simulink model "satellite_attitude_kalman_model"  (R2017a)
settings: Solver=VariableStepAuto  StartTime=0.0  StopTime=tdur  FixedStep=dt  RelTol=1e-3
values from neighbouring files (symbols this model uses):
  Ad_b = expm(A_b*dt)    [linear_eq.m]
  Ad_rw = sysd_rw.a    [satellite_attitude_kalman_run.m]
  b = 0.000178    [satellite_attitude_kalman_run.m]
  Bd_b = integral(fun,0,dt,'ArrayValued',true)*B_b    [linear_eq.m]
  Bd_rw = sysd_rw.b    [satellite_attitude_kalman_run.m]
  C_lqe = [ 0 0 0 0 0 0 ... (first row only)    [satellite_attitude_kalman_run.m]
  Cd_rw = sysd_rw.c    [satellite_attitude_kalman_run.m]
  DCM_b_i_0 = eul2qua(x_pos_init,y_pos_init,z_pos_init)    [satellite_attitude_kalman_run.m]
  DCM_b_w = [ 0.40825 0.40825 -0.81650 ... (first row only)    [satellite_attitude_kalman_run.m]
  dt_c = 0.05    [satellite_attitude_kalman_run.m]
  dt_w = 0.05    [satellite_attitude_kalman_run.m]
  grav_ref = [0 ; 0 ; -1]    [satellite_attitude_kalman_run.m]
  grav_variance = 0    [satellite_attitude_kalman_run.m]
  i_0 = [0 ;0 ;0]    [satellite_attitude_kalman_run.m]
  I_b = diag([Ixx Iyy Izz])    [satellite_attitude_kalman_run.m]
  I_w = diag([Ia Ia Ia])    [satellite_attitude_kalman_run.m]
  J = 0.00725    [satellite_attitude_kalman_run.m]
  K_e = 0.071    [satellite_attitude_kalman_run.m]
  K_t = 0.070    (= 0.07)    [satellite_attitude_kalman_run.m]
  Kd = 1.5    [satellite_attitude_kalman_run.m]
  Kp = dlqr(Ad_b,Bd_b,Q_lqr,R_lqr)    [satellite_attitude_kalman_run.m]
  L = 0.00339    [satellite_attitude_kalman_run.m]
  Lss = dlqe(Ad_b, eye(6,6),C_lqe, Q_lqe,R_lqe)    [satellite_attitude_kalman_run.m]
  mag_ref = [0 ; 1400 ; 0]    [satellite_attitude_kalman_run.m]
  mag_variance = [0;0;0]    [satellite_attitude_kalman_run.m]
  omega_0 = [x_rate_init ;y_rate_init ;z_rate_init]    [satellite_attitude_kalman_run.m]
  omega_variance = [0;0;0]    [satellite_attitude_kalman_run.m]
  R = 1.52    [satellite_attitude_kalman_run.m]
  speed_0 = [RW1_init ;RW2_init ;RW3_init]    [satellite_attitude_kalman_run.m]
  theta_0 = [x_pos_init ;y_pos_init ;z_pos_init]    [satellite_attitude_kalman_run.m]
  v_max = 10    [satellite_attitude_kalman_run.m]
undefined symbols (not defined in the file or in its folder): DiscIntNeverNeededParam
libraries: simulink x20, vrlib x6, dspinverses x3
settings Model: Creator=Goh  LastModifiedBy=Rusty Goh
settings SolverCC: MaxConsecutiveMinStep=2

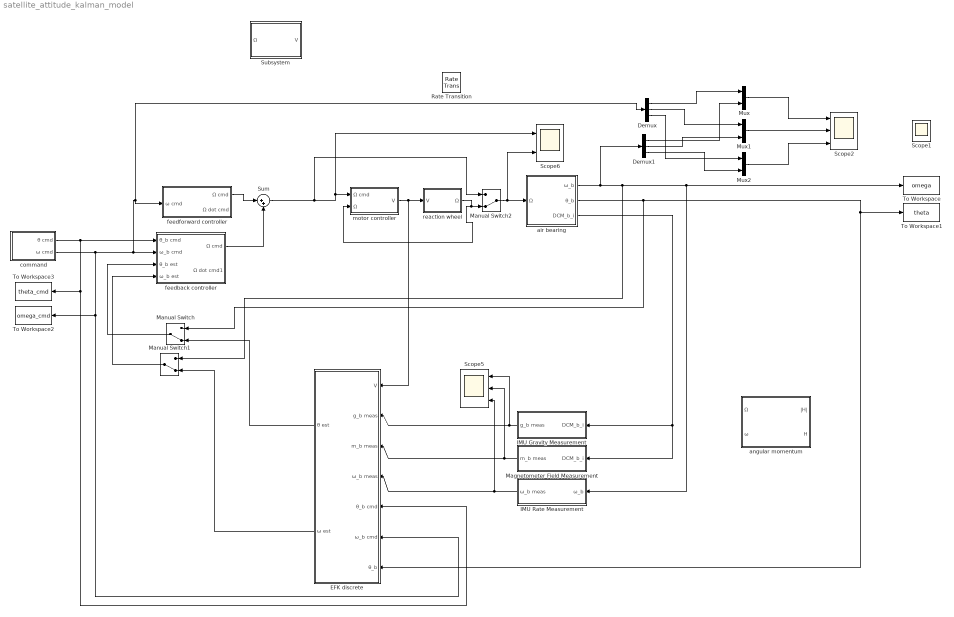
== system satellite_attitude_kalman_model ==
  Demux : Demux  Outputs=3
  Demux1 : Demux  Outputs=3
  EFK discrete : Subsystem
  IMU Gravity Measurement : Subsystem
  IMU Rate Measurement : Subsystem
  Magnetometer Field Measurement : Subsystem
  Manual Switch : ManualSwitch  CurrentSetting=0
  Manual Switch1 : ManualSwitch  CurrentSetting=0
  Manual Switch2 : ManualSwitch  CurrentSetting=0
  Mux : Mux  Inputs=2
  Mux1 : Mux  Inputs=2
  Mux2 : Mux  Inputs=2
  Rate Transition : RateTransition
  Scope1 : Scope  NumInputPorts=3
  Scope2 : Scope  NumInputPorts=3
  Scope5 : Scope  NumInputPorts=3
  Scope6 : Scope  NumInputPorts=2
  Subsystem : Subsystem  mask{Kc=1, Kp=75, Ki=1, Kd=1}
  Sum : Sum  Inputs=|++
  To Workspace : ToWorkspace  VariableName=omega  SampleTime=-1
  To Workspace1 : ToWorkspace  VariableName=theta  SampleTime=-1
  To Workspace2 : ToWorkspace  VariableName=omega_cmd  SaveFormat=Timeseries  SampleTime=-1
  To Workspace3 : ToWorkspace  VariableName=theta_cmd  SaveFormat=Timeseries  SampleTime=-1
  air bearing : Subsystem
  angular momentum : Subsystem
  command : Subsystem
  feedback controller : Subsystem
  feedforward controller : Subsystem
  motor controller : Subsystem
  reaction wheel : Subsystem
  wires:
  Magnetometer Field Measurement/1(m_b meas) -> Scope5/2, EFK discrete/3(m_b meas)
  IMU Rate Measurement/1(ω_b meas) -> Scope5/3, EFK discrete/4(ω_b meas)
  IMU Gravity Measurement/1(g_b meas) -> Scope5/1, EFK discrete/2(g_b meas)
  command/1(θ cmd) -> To Workspace3/1, EFK discrete/5(θ_b cmd), feedback controller/1(θ_b cmd)
  feedback controller/1(Ω cmd) -> Sum/2
  command/2(ω cmd) -> To Workspace2/1, EFK discrete/6(ω_b cmd), Demux/1, feedforward controller/1(ω cmd), feedback controller/2(ω_b cmd)
  air bearing/2(θ_b) -> Manual Switch/1, To Workspace1/1, EFK discrete/7("θ_b ")
  feedforward controller/1(Ω cmd) -> Sum/1
  Mux/1 -> Scope2/1
  Mux1/1 -> Scope2/2
  Mux2/1 -> Scope2/3
  Demux/1 -> Mux/1
  Demux1/1 -> Mux/2
  Demux/2 -> Mux1/1
  Demux1/2 -> Mux1/2
  Demux/3 -> Mux2/1
  Demux1/3 -> Mux2/2
  air bearing/3(DCM_b_i) -> Magnetometer Field Measurement/1(DCM_b_i), IMU Gravity Measurement/1(DCM_b_i)
  EFK discrete/2(ω est) -> Manual Switch1/2
  air bearing/1(ω_b) -> Demux1/1, Manual Switch1/1, IMU Rate Measurement/1(ω_b), To Workspace/1
  EFK discrete/1(θ est) -> Manual Switch/2
  Manual Switch/1 -> feedback controller/3(θ_b est)
  Manual Switch1/1 -> feedback controller/4(ω_b est)
  motor controller/1(V) -> EFK discrete/1(V), reaction wheel/1(V)
  Manual Switch2/1 -> Scope6/2, air bearing/1(Ω)
  reaction wheel/1(Ω) -> Manual Switch2/2, motor controller/2(Ω)
  Sum/1 -> Manual Switch2/1, motor controller/1(Ω cmd), Scope6/1

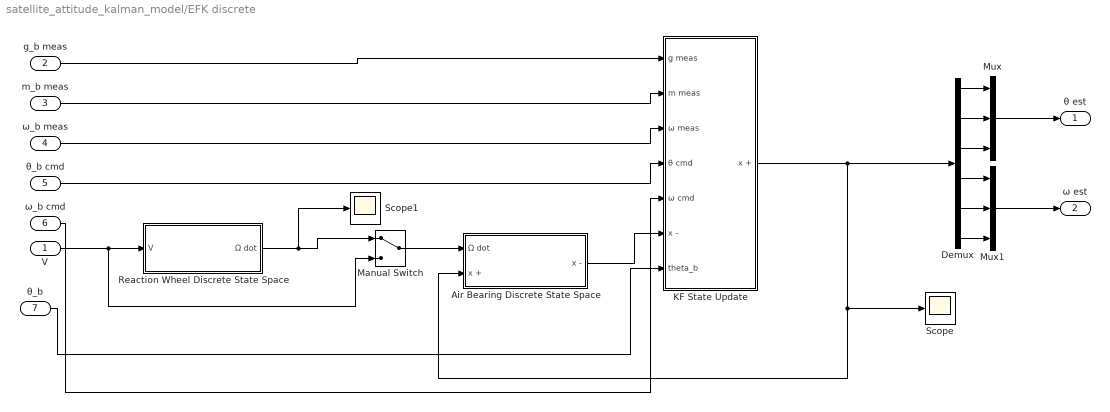
== system satellite_attitude_kalman_model/EFK discrete ==
  V : Inport
  g_b meas : Inport  Port=2
  m_b meas : Inport  Port=3
  ω_b meas : Inport  Port=4
  θ_b cmd : Inport  Port=5
  ω_b cmd : Inport  Port=6
  "θ_b " : Inport  Port=7
  Air Bearing Discrete State Space : Subsystem
  Demux : Demux  Outputs=6
  KF State Update : Subsystem
  Manual Switch : ManualSwitch
  Mux : Mux  Inputs=3
  Mux1 : Mux  Inputs=3
  Reaction Wheel Discrete State Space : Subsystem
  Scope : Scope
  Scope1 : Scope
  θ est : Outport
  ω est : Outport  Port=2
  wires:
  g_b meas/1 -> KF State Update/1(g meas)
  m_b meas/1 -> KF State Update/2(m meas)
  ω_b meas/1 -> KF State Update/3(ω meas)
  θ_b cmd/1 -> KF State Update/4(θ cmd)
  ω_b cmd/1 -> KF State Update/5(ω cmd)
  Air Bearing Discrete State Space/1(x -) -> KF State Update/6(x -)
  Demux/2 -> Mux/2
  Demux/1 -> Mux/1
  Demux/3 -> Mux/3
  Demux/4 -> Mux1/1
  Demux/5 -> Mux1/2
  Demux/6 -> Mux1/3
  Mux/1 -> θ est/1
  Mux1/1 -> ω est/1
  "θ_b "/1 -> KF State Update/7(theta_b)
  KF State Update/1(x +) -> Air Bearing Discrete State Space/2(x +), Scope/1, Demux/1
  V/1 -> Reaction Wheel Discrete State Space/1(V), Manual Switch/2
  Manual Switch/1 -> Air Bearing Discrete State Space/1(Ω dot)
  Reaction Wheel Discrete State Space/1(Ω dot) -> Scope1/1, Manual Switch/1

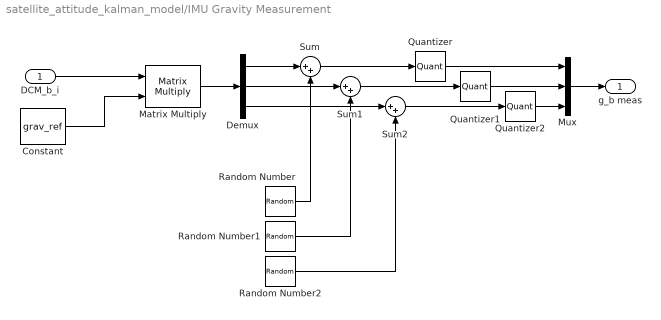
== system satellite_attitude_kalman_model/IMU Gravity Measurement ==
  DCM_b_i : Inport
  Constant : Constant  Value=grav_ref  VectorParams1D=off
  Demux : Demux  Outputs=3
  Matrix Multiply : Product  Multiplication=Matrix(*)
  Mux : Mux  Inputs=3
  Quantizer : Quantizer  QuantizationInterval=0.01
  Quantizer1 : Quantizer  QuantizationInterval=0.01
  Quantizer2 : Quantizer  QuantizationInterval=0.01
  Random Number : RandomNumber  Variance=grav_variance  SampleTime=dt_c
  Random Number1 : RandomNumber  Variance=grav_variance  SampleTime=dt_c
  Random Number2 : RandomNumber  Variance=grav_variance  SampleTime=dt_c
  Sum : Sum  Inputs=|++
  Sum1 : Sum  Inputs=|++
  Sum2 : Sum  Inputs=|++
  g_b meas : Outport
  wires:
  Demux/1 -> Sum/1
  Demux/2 -> Sum1/1
  Demux/3 -> Sum2/1
  Sum2/1 -> Quantizer2/1
  Sum1/1 -> Quantizer1/1
  Sum/1 -> Quantizer/1
  Random Number/1 -> Sum/2
  Random Number1/1 -> Sum1/2
  Random Number2/1 -> Sum2/2
  Mux/1 -> g_b meas/1
  DCM_b_i/1 -> Matrix Multiply/1
  Constant/1 -> Matrix Multiply/2
  Matrix Multiply/1 -> Demux/1
  Quantizer/1 -> Mux/1
  Quantizer1/1 -> Mux/2
  Quantizer2/1 -> Mux/3

== system satellite_attitude_kalman_model/IMU Rate Measurement ==
  ω_b : Inport
  Demux : Demux  Outputs=3
  Mux : Mux  Inputs=3
  Random Number : RandomNumber  Variance=omega_variance(1)  SampleTime=dt_c
  Random Number1 : RandomNumber  Variance=omega_variance(2)  SampleTime=dt_c
  Random Number2 : RandomNumber  Variance=omega_variance(3)  SampleTime=dt_c
  Sum : Sum  Inputs=|++
  Sum1 : Sum  Inputs=|++
  Sum2 : Sum  Inputs=|++
  Zero-Order Hold : ZeroOrderHold  SampleTime=dt_c
  ω_b meas : Outport
  wires:
  Demux/1 -> Sum/1
  Demux/2 -> Sum1/1
  Demux/3 -> Sum2/1
  Sum2/1 -> Mux/3
  Sum1/1 -> Mux/2
  Sum/1 -> Mux/1
  Random Number/1 -> Sum/2
  Random Number1/1 -> Sum1/2
  Random Number2/1 -> Sum2/2
  Mux/1 -> ω_b meas/1
  ω_b/1 -> Zero-Order Hold/1
  Zero-Order Hold/1 -> Demux/1

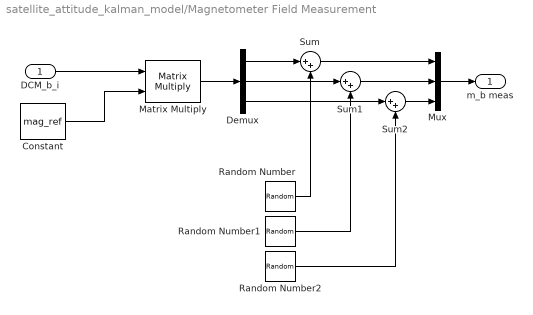
== system satellite_attitude_kalman_model/Magnetometer Field Measurement ==
  DCM_b_i : Inport
  Constant : Constant  Value=mag_ref  VectorParams1D=off
  Demux : Demux  Outputs=3
  Matrix Multiply : Product  Multiplication=Matrix(*)
  Mux : Mux  Inputs=3
  Random Number : RandomNumber  Variance=mag_variance(1)  SampleTime=dt_c
  Random Number1 : RandomNumber  Variance=mag_variance(2)  SampleTime=dt_c
  Random Number2 : RandomNumber  Variance=mag_variance(3)  SampleTime=dt_c
  Sum : Sum  Inputs=|++
  Sum1 : Sum  Inputs=|++
  Sum2 : Sum  Inputs=|++
  m_b meas : Outport
  wires:
  Demux/1 -> Sum/1
  Demux/2 -> Sum1/1
  Demux/3 -> Sum2/1
  Sum2/1 -> Mux/3
  Sum1/1 -> Mux/2
  Sum/1 -> Mux/1
  Random Number/1 -> Sum/2
  Random Number1/1 -> Sum1/2
  Random Number2/1 -> Sum2/2
  Mux/1 -> m_b meas/1
  DCM_b_i/1 -> Matrix Multiply/1
  Constant/1 -> Matrix Multiply/2
  Matrix Multiply/1 -> Demux/1

== system satellite_attitude_kalman_model/Subsystem ==
  Ω : Inport
  Discrete Derivative : simulink/Discrete/Discrete Derivative  gainval=1.0  ICPrevScaledInput=0.0  OutMin=[]  OutMax=[]  OutDataType=fixdt(1, 16)  OutScaling=2^-10  DoSatur=off
  Discrete-Time Integrator : DiscreteIntegrator  InitialConditionSetting=State (most efficient)  SampleTime=-1  ICPrevOutput=DiscIntNeverNeededParam  ICPrevScaledInput=DiscIntNeverNeededParam
  Kc : Gain  Gain=Kc  SaturateOnIntegerOverflow=on  OutDataTypeStr=Inherit: Same as input  ParamDataTypeStr=Inherit: Same as input
  Kd : Gain  Gain=Kd  SaturateOnIntegerOverflow=on  OutDataTypeStr=Inherit: Same as input  ParamDataTypeStr=Inherit: Same as input
  Ki : Gain  Gain=Ki  SaturateOnIntegerOverflow=on  OutDataTypeStr=Inherit: Same as input  ParamDataTypeStr=Inherit: Same as input
  Kp : Gain  Gain=Kp  SaturateOnIntegerOverflow=on  OutDataTypeStr=Inherit: Same as input  ParamDataTypeStr=Inherit: Same as input
  Sum1 : Sum  Inputs=+++
  V : Outport
  wires:
  Ki/1 -> Discrete-Time Integrator/1
  Kc/1 -> Ki/1, Kp/1, Kd/1
  Sum1/1 -> V/1
  Kd/1 -> Discrete Derivative/1
  Discrete Derivative/1 -> Sum1/1
  Kp/1 -> Sum1/2
  Discrete-Time Integrator/1 -> Sum1/3
  Ω/1 -> Kc/1

== system satellite_attitude_kalman_model/air bearing ==
  Ω : Inport
  Integrator : Integrator  InitialCondition=omega_0
  Integrator1 : Integrator  InitialCondition=theta_0
  air bearing dyamics : Subsystem
  ω to DCM : Subsystem
  ω_b : Outport
  θ_b : Outport  Port=2
  DCM_b_i : Outport  Port=3
  wires:
  Ω/1 -> air bearing dyamics/1(Ω_w)
  air bearing dyamics/1(ω_dot) -> Integrator/1
  Integrator/1 -> ω to DCM/1(ω), ω_b/1, Integrator1/1, air bearing dyamics/2(ω_b)
  Integrator1/1 -> θ_b/1
  ω to DCM/1(DCM_b_i) -> DCM_b_i/1

== system satellite_attitude_kalman_model/angular momentum ==
  Ω : Inport
  ω : Inport  Port=2
  |H| : Outport
  H : Outport  Port=2

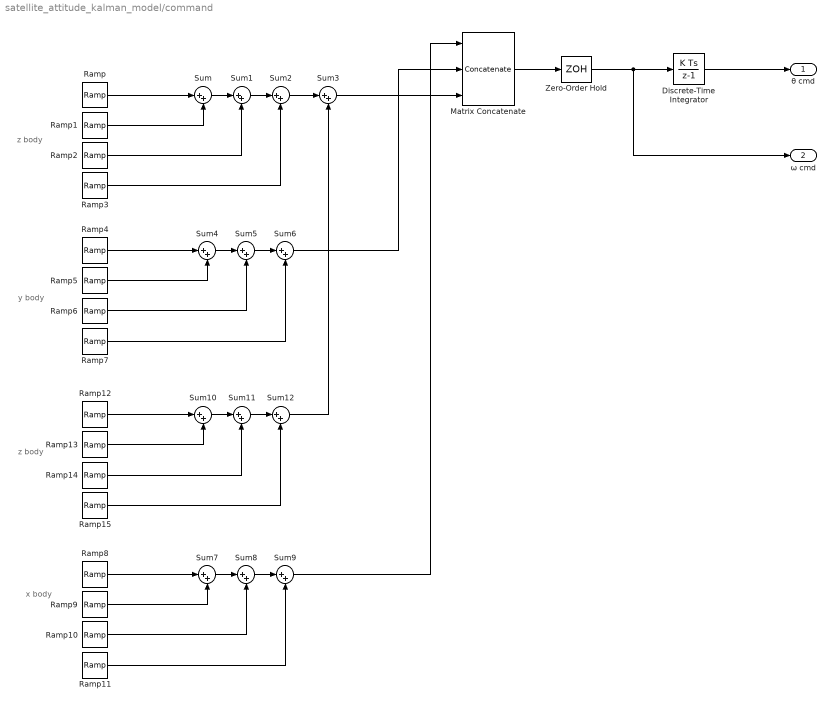
== system satellite_attitude_kalman_model/command ==
  note: x body
  note: z body
  note: y body
  note: z body
  Discrete-Time Integrator : DiscreteIntegrator  SampleTime=dt_c  ICPrevOutput=DiscIntNeverNeededParam  ICPrevScaledInput=DiscIntNeverNeededParam
  Matrix Concatenate : Concatenate  NumInputs=3  Mode=Multidimensional array
  Ramp : simulink/Sources/Ramp  slope=0.01  start=5  X0=0
  Ramp1 : simulink/Sources/Ramp  slope=-0.01  start=15  X0=0
  Ramp10 : simulink/Sources/Ramp  slope=-0.005  start=195  X0=0
  Ramp11 : simulink/Sources/Ramp  slope=0.005  start=205  X0=0
  Ramp12 : simulink/Sources/Ramp  slope=-0.01  start=125  X0=0
  Ramp13 : simulink/Sources/Ramp  slope=0.01  start=135  X0=0
  Ramp14 : simulink/Sources/Ramp  slope=0.01  start=145  X0=0
  Ramp15 : simulink/Sources/Ramp  slope=-0.01  start=155  X0=0
  Ramp2 : simulink/Sources/Ramp  slope=-0.01  start=25  X0=0
  Ramp3 : simulink/Sources/Ramp  slope=0.01  start=35  X0=0
  Ramp4 : simulink/Sources/Ramp  slope=0.005  start=55  X0=0
  Ramp5 : simulink/Sources/Ramp  slope=-0.005  start=65  X0=0
  Ramp6 : simulink/Sources/Ramp  slope=-0.005  start=75  X0=0
  Ramp7 : simulink/Sources/Ramp  slope=0.005  start=85  X0=0
  Ramp8 : simulink/Sources/Ramp  slope=0.005  start=175  X0=0
  Ramp9 : simulink/Sources/Ramp  slope=-0.005  start=185  X0=0
  Sum{,1..12} (13 alike) : Sum  Inputs=|++
  Zero-Order Hold : ZeroOrderHold  SampleTime=dt_c
  θ cmd : Outport
  ω cmd : Outport  Port=2
  wires:
  Sum/1 -> Sum1/1
  Sum1/1 -> Sum2/1
  Sum4/1 -> Sum5/1
  Sum5/1 -> Sum6/1
  Sum7/1 -> Sum8/1
  Sum8/1 -> Sum9/1
  Ramp/1 -> Sum/1
  Ramp2/1 -> Sum1/2
  Ramp3/1 -> Sum2/2
  Ramp4/1 -> Sum4/1
  Ramp5/1 -> Sum4/2
  Ramp6/1 -> Sum5/2
  Ramp7/1 -> Sum6/2
  Ramp8/1 -> Sum7/1
  Ramp9/1 -> Sum7/2
  Ramp10/1 -> Sum8/2
  Ramp11/1 -> Sum9/2
  Sum6/1 -> Matrix Concatenate/2
  Matrix Concatenate/1 -> Zero-Order Hold/1
  Zero-Order Hold/1 -> ω cmd/1, Discrete-Time Integrator/1
  Discrete-Time Integrator/1 -> θ cmd/1
  Ramp1/1 -> Sum/2
  Sum3/1 -> Matrix Concatenate/3
  Sum2/1 -> Sum3/1
  Sum9/1 -> Matrix Concatenate/1
  Sum10/1 -> Sum11/1
  Sum11/1 -> Sum12/1
  Ramp12/1 -> Sum10/1
  Ramp14/1 -> Sum11/2
  Ramp15/1 -> Sum12/2
  Ramp13/1 -> Sum10/2
  Sum12/1 -> Sum3/2

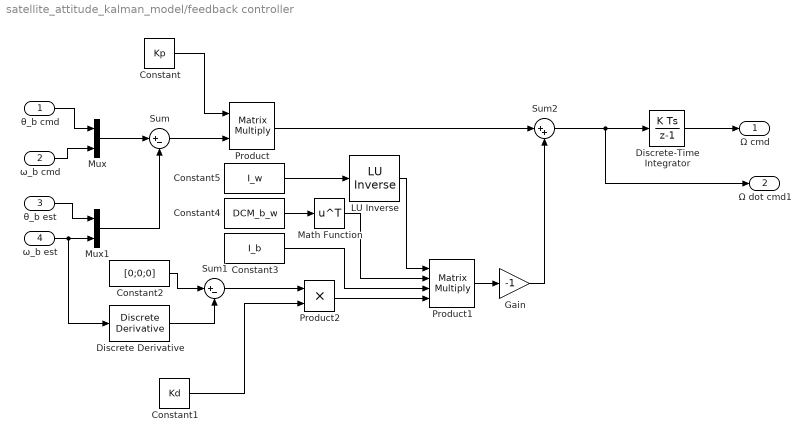
== system satellite_attitude_kalman_model/feedback controller ==
  θ_b cmd : Inport
  ω_b cmd : Inport  Port=2
  θ_b est : Inport  Port=3
  ω_b est : Inport  Port=4
  " LU Inverse" : dspinverses/ LU Inverse
      settings: SourceProductName=DSP System Toolbox
  Constant : Constant  Value=Kp  VectorParams1D=off
  Constant1 : Constant  Value=Kd
  Constant2 : Constant  Value=[0;0;0]  VectorParams1D=off
  Constant3 : Constant  Value=I_b
  Constant4 : Constant  Value=DCM_b_w  VectorParams1D=off
  Constant5 : Constant  Value=I_w  VectorParams1D=off
  Discrete Derivative : simulink/Discrete/Discrete Derivative  gainval=1.0  ICPrevScaledInput=0.0  OutMin=[]  OutMax=[]  OutDataType=fixdt(1, 16)  OutScaling=2^-10  DoSatur=off
  Discrete-Time Integrator : DiscreteIntegrator  InitialConditionSetting=State (most efficient)  SampleTime=dt_c  ICPrevOutput=DiscIntNeverNeededParam  ICPrevScaledInput=DiscIntNeverNeededParam
  Gain : Gain  Gain=-1
  Math Function : Math  Operator=transpose  SaturateOnIntegerOverflow=on
  Mux : Mux  Inputs=2
  Mux1 : Mux  Inputs=2
  Product : Product  Multiplication=Matrix(*)
  Product1 : Product  Inputs=4  Multiplication=Matrix(*)
  Product2 : Product
  Sum : Sum  Inputs=|+-
  Sum1 : Sum  Inputs=|+-
  Sum2 : Sum  Inputs=|++
  Ω cmd : Outport
  Ω dot cmd1 : Outport  Port=2
  wires:
  ω_b cmd/1 -> Mux/2
  θ_b cmd/1 -> Mux/1
  θ_b est/1 -> Mux1/1
  ω_b est/1 -> Discrete Derivative/1, Mux1/2
  Mux/1 -> Sum/1
  Mux1/1 -> Sum/2
  Sum/1 -> Product/2
  Constant/1 -> Product/1
  Product2/1 -> Product1/4
  Constant1/1 -> Product2/2
  Sum1/1 -> Product2/1
  Discrete Derivative/1 -> Sum1/2
  Constant2/1 -> Sum1/1
  Sum2/1 -> Ω dot cmd1/1, Discrete-Time Integrator/1
  Discrete-Time Integrator/1 -> Ω cmd/1
  Product1/1 -> Gain/1
  Gain/1 -> Sum2/2
  Product/1 -> Sum2/1
  Constant3/1 -> Product1/3
  Constant5/1 -> " LU Inverse"/1
  Constant4/1 -> Math Function/1
  " LU Inverse"/1 -> Product1/1
  Math Function/1 -> Product1/2

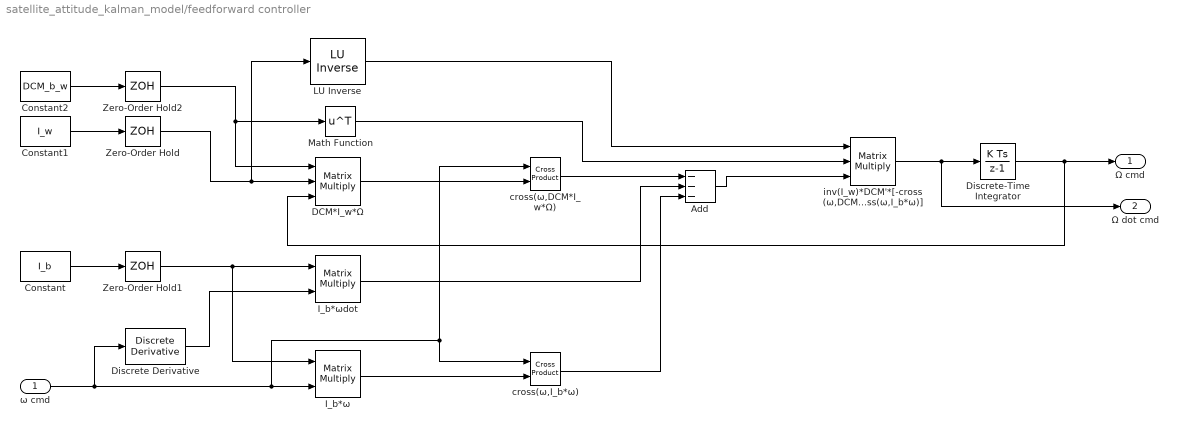
== system satellite_attitude_kalman_model/feedforward controller ==
  ω cmd : Inport
  " LU Inverse" : dspinverses/ LU Inverse
      settings: SourceProductName=DSP System Toolbox
  Add : Sum  Inputs=---
  Constant : Constant  Value=I_b  VectorParams1D=off  SampleTime=-1
  Constant1 : Constant  Value=I_w  VectorParams1D=off  SampleTime=-1
  Constant2 : Constant  Value=DCM_b_w  VectorParams1D=off  SampleTime=-1
  DCM*I_w*Ω : Product  Inputs=3  Multiplication=Matrix(*)
  Discrete Derivative : simulink/Discrete/Discrete Derivative  gainval=1.0  ICPrevScaledInput=0.0  OutMin=[]  OutMax=[]  OutDataType=fixdt(1, 16)  OutScaling=2^-10  DoSatur=off
  Discrete-Time Integrator : DiscreteIntegrator  gainval=1  SampleTime=dt_c  ICPrevOutput=DiscIntNeverNeededParam  ICPrevScaledInput=DiscIntNeverNeededParam
  I_b*ω : Product  Multiplication=Matrix(*)
  I_b*ωdot : Product  Multiplication=Matrix(*)
  Math Function : Math  Operator=transpose  SaturateOnIntegerOverflow=on
  Zero-Order Hold : ZeroOrderHold  SampleTime=dt_c
  Zero-Order Hold1 : ZeroOrderHold  SampleTime=dt_c
  Zero-Order Hold2 : ZeroOrderHold  SampleTime=dt_c
  cross(ω,DCM*I_w*Ω) : vrlib/Utilities/Cross Product
      settings: SourceProductBaseCode=VR
  cross(ω,I_b*ω) : vrlib/Utilities/Cross Product
      settings: SourceProductBaseCode=VR
  inv(I_w)*DCM'*[-cross(ω,DCM*I_w*Ω)-I_b*ωdot-cross(ω,I_b*ω)] : Product  Inputs=3  Multiplication=Matrix(*)
  Ω cmd : Outport
  Ω dot cmd : Outport  Port=2
  wires:
  ω cmd/1 -> Discrete Derivative/1, I_b*ω/2, cross(ω,I_b*ω)/1, cross(ω,DCM*I_w*Ω)/1
  DCM*I_w*Ω/1 -> cross(ω,DCM*I_w*Ω)/2
  cross(ω,DCM*I_w*Ω)/1 -> Add/1
  I_b*ω/1 -> cross(ω,I_b*ω)/2
  inv(I_w)*DCM'*[-cross(ω,DCM*I_w*Ω)-I_b*ωdot-cross(ω,I_b*ω)]/1 -> Ω dot cmd/1, Discrete-Time Integrator/1
  Add/1 -> inv(I_w)*DCM'*[-cross(ω,DCM*I_w*Ω)-I_b*ωdot-cross(ω,I_b*ω)]/3
  " LU Inverse"/1 -> inv(I_w)*DCM'*[-cross(ω,DCM*I_w*Ω)-I_b*ωdot-cross(ω,I_b*ω)]/1
  Constant2/1 -> Zero-Order Hold2/1
  Constant1/1 -> Zero-Order Hold/1
  Discrete Derivative/1 -> I_b*ωdot/2
  Constant/1 -> Zero-Order Hold1/1
  I_b*ωdot/1 -> Add/2
  cross(ω,I_b*ω)/1 -> Add/3
  Discrete-Time Integrator/1 -> Ω cmd/1, DCM*I_w*Ω/3
  Math Function/1 -> inv(I_w)*DCM'*[-cross(ω,DCM*I_w*Ω)-I_b*ωdot-cross(ω,I_b*ω)]/2
  Zero-Order Hold1/1 -> I_b*ω/1, I_b*ωdot/1
  Zero-Order Hold/1 -> " LU Inverse"/1, DCM*I_w*Ω/2
  Zero-Order Hold2/1 -> DCM*I_w*Ω/1, Math Function/1

== system satellite_attitude_kalman_model/motor controller ==
  Ω cmd : Inport
  Ω : Inport  Port=2
  Constant1 : Constant  Value=-v_max
  Constant2 : Constant  Value=v_max
  Relational Operator : RelationalOperator  Operator=>  OutDataTypeStr=boolean  RndMeth=Simplest
  Switch : Switch  Criteria=u2 > Threshold
  Zero-Order Hold : ZeroOrderHold  SampleTime=dt_c
  V : Outport
  wires:
  Switch/1 -> Zero-Order Hold/1
  Relational Operator/1 -> Switch/2
  Zero-Order Hold/1 -> V/1
  Ω cmd/1 -> Relational Operator/1
  Ω/1 -> Relational Operator/2
  Constant1/1 -> Switch/3
  Constant2/1 -> Switch/1

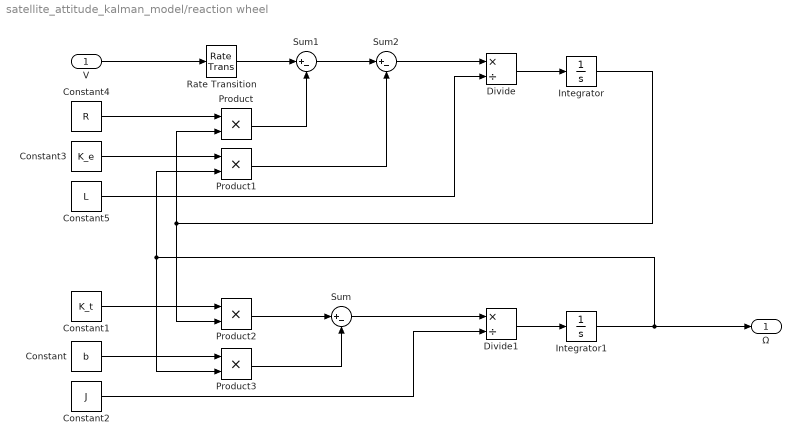
== system satellite_attitude_kalman_model/reaction wheel ==
  V : Inport
  Constant : Constant  Value=b
  Constant1 : Constant  Value=K_t  VectorParams1D=off
  Constant2 : Constant  Value=J
  Constant3 : Constant  Value=K_e  VectorParams1D=off
  Constant4 : Constant  Value=R
  Constant5 : Constant  Value=L
  Divide : Product  Inputs=*/
  Divide1 : Product  Inputs=*/
  Integrator : Integrator  InitialCondition=i_0
  Integrator1 : Integrator  InitialCondition=speed_0
  Product{,1..3} (4 alike) : Product
  Rate Transition : RateTransition
  Sum : Sum  Inputs=|+-
  Sum1 : Sum  Inputs=|+-
  Sum2 : Sum  Inputs=|+-
  Ω : Outport
  wires:
  Product2/1 -> Sum/1
  Product3/1 -> Sum/2
  Product/1 -> Sum1/2
  Sum1/1 -> Sum2/1
  Product1/1 -> Sum2/2
  Sum2/1 -> Divide/1
  Divide/1 -> Integrator/1
  Sum/1 -> Divide1/1
  Divide1/1 -> Integrator1/1
  Integrator1/1 -> Product3/2, Product1/2, Ω/1
  Constant3/1 -> Product1/1
  Constant4/1 -> Product/1
  Constant5/1 -> Divide/2
  Integrator/1 -> Product/2, Product2/2
  Constant2/1 -> Divide1/2
  Constant/1 -> Product3/1
  Constant1/1 -> Product2/1
  V/1 -> Rate Transition/1
  Rate Transition/1 -> Sum1/1

== system satellite_attitude_kalman_model/EFK discrete/Air Bearing Discrete State Space ==
  Ω dot : Inport
  x + : Inport  Port=2
  Constant : Constant  Value=Bd_b  VectorParams1D=off  SampleTime=dt_c
  Constant1 : Constant  Value=Ad_b  VectorParams1D=off  SampleTime=dt_c
  Matrix Multiply : Product  Multiplication=Matrix(*)
  Matrix Multiply1 : Product  Multiplication=Matrix(*)
  Sum : Sum  Inputs=|++
  x - : Outport
  wires:
  Constant1/1 -> Matrix Multiply1/1
  x +/1 -> Matrix Multiply1/2
  Ω dot/1 -> Matrix Multiply/2
  Sum/1 -> x -/1
  Matrix Multiply1/1 -> Sum/2
  Constant/1 -> Matrix Multiply/1
  Matrix Multiply/1 -> Sum/1

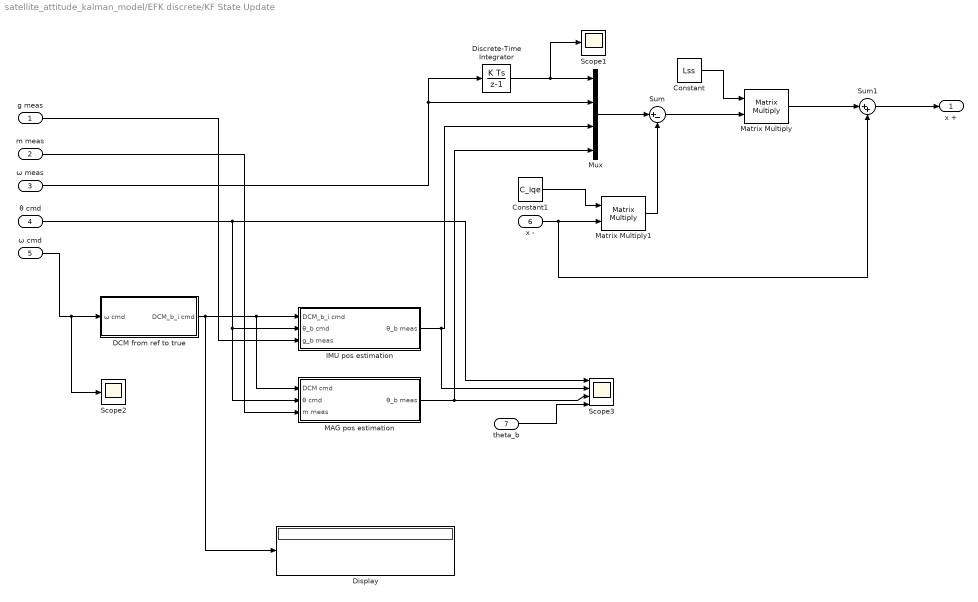
== system satellite_attitude_kalman_model/EFK discrete/KF State Update ==
  g meas : Inport
  m meas : Inport  Port=2
  ω meas : Inport  Port=3
  θ cmd : Inport  Port=4
  ω cmd : Inport  Port=5
  x - : Inport  Port=6
  theta_b : Inport  Port=7
  Constant : Constant  Value=Lss  VectorParams1D=off  SampleTime=dt_c
  Constant1 : Constant  Value=C_lqe  VectorParams1D=off  SampleTime=dt_c
  DCM from ref to true : Subsystem
  Discrete-Time Integrator : DiscreteIntegrator  InitialConditionSetting=State (most efficient)  SampleTime=dt_c  ICPrevOutput=DiscIntNeverNeededParam  ICPrevScaledInput=DiscIntNeverNeededParam
  Display : Display
  IMU pos estimation : Subsystem
  MAG pos estimation : Subsystem
  Matrix Multiply : Product  Multiplication=Matrix(*)
  Matrix Multiply1 : Product  Multiplication=Matrix(*)
  Mux : Mux
  Scope1 : Scope
  Scope2 : Scope
  Scope3 : Scope  NumInputPorts=4
  Sum : Sum  Inputs=|+-
  Sum1 : Sum  Inputs=|++
  x + : Outport
  wires:
  MAG pos estimation/1(θ_b meas) -> Scope3/3, Mux/4
  Discrete-Time Integrator/1 -> Scope1/1, Mux/1
  Constant/1 -> Matrix Multiply/1
  Constant1/1 -> Matrix Multiply1/1
  DCM from ref to true/1(DCM_b_i cmd) -> Display/1, MAG pos estimation/1(DCM cmd), IMU pos estimation/1(DCM_b_i cmd)
  Sum/1 -> Matrix Multiply/2
  ω meas/1 -> Discrete-Time Integrator/1, Mux/2
  Sum1/1 -> x +/1
  x -/1 -> Sum1/2, Matrix Multiply1/2
  Matrix Multiply1/1 -> Sum/2
  ω cmd/1 -> Scope2/1, DCM from ref to true/1(ω cmd)
  IMU pos estimation/1(θ_b meas) -> Scope3/2, Mux/3
  m meas/1 -> MAG pos estimation/3(m meas)
  Matrix Multiply/1 -> Sum1/1
  Mux/1 -> Sum/1
  g meas/1 -> IMU pos estimation/3(g_b meas)
  θ cmd/1 -> Scope3/1, MAG pos estimation/2(θ cmd), IMU pos estimation/2(θ_b cmd)
  theta_b/1 -> Scope3/4

== system satellite_attitude_kalman_model/EFK discrete/Reaction Wheel Discrete State Space ==
  V : Inport
  Constant : Constant  Value=Cd_rw  VectorParams1D=off
  Constant1 : Constant  Value=Ad_rw  VectorParams1D=off
  Constant2 : Constant  Value=Bd_rw  VectorParams1D=off
  Discrete Derivative : simulink/Discrete/Discrete Derivative  gainval=1.0  ICPrevScaledInput=0.0  OutMin=[]  OutMax=[]  OutDataType=fixdt(1, 16)  OutScaling=2^-10  DoSatur=off
  Matrix Multiply : Product  Multiplication=Matrix(*)
  Matrix Multiply1 : Product  Multiplication=Matrix(*)
  Matrix Multiply2 : Product  Multiplication=Matrix(*)
  Sum : Sum  Inputs=|++
  Unit Delay : UnitDelay  SampleTime=dt_c
  Ω dot : Outport
  wires:
  Matrix Multiply/1 -> Sum/1
  Sum/1 -> Matrix Multiply1/2, Unit Delay/1
  Constant2/1 -> Matrix Multiply/1
  Matrix Multiply2/1 -> Sum/2
  Matrix Multiply1/1 -> Discrete Derivative/1
  Discrete Derivative/1 -> Ω dot/1
  Constant/1 -> Matrix Multiply1/1
  Constant1/1 -> Matrix Multiply2/1
  Unit Delay/1 -> Matrix Multiply2/2
  V/1 -> Matrix Multiply/2

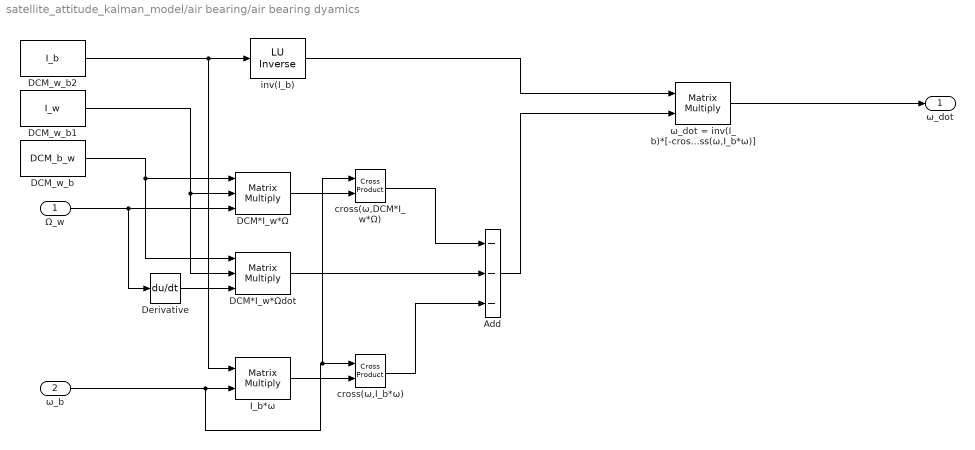
== system satellite_attitude_kalman_model/air bearing/air bearing dyamics ==
  Ω_w : Inport
  ω_b : Inport  Port=2
  Add : Sum  Inputs=---
  DCM*I_w*Ω : Product  Inputs=3  Multiplication=Matrix(*)
  DCM*I_w*Ωdot : Product  Inputs=3  Multiplication=Matrix(*)
  DCM_w_b : Constant  Value=DCM_b_w  VectorParams1D=off
  DCM_w_b1 : Constant  Value=I_w  VectorParams1D=off
  DCM_w_b2 : Constant  Value=I_b  VectorParams1D=off
  Derivative : Derivative
  I_b*ω : Product  Multiplication=Matrix(*)
  cross(ω,DCM*I_w*Ω) : vrlib/Utilities/Cross Product
      settings: SourceProductBaseCode=VR
  cross(ω,I_b*ω) : vrlib/Utilities/Cross Product
      settings: SourceProductBaseCode=VR
  inv(I_b) : dspinverses/ LU Inverse
      settings: SourceProductName=DSP System Toolbox
  ω_dot = inv(I_b)*[-cross(ω,DCM*I_w*Ω)-DCM*I_w*Ωdot-cross(ω,I_b*ω)] : Product  Multiplication=Matrix(*)
  ω_dot : Outport
  wires:
  Derivative/1 -> DCM*I_w*Ωdot/3
  Ω_w/1 -> Derivative/1, DCM*I_w*Ω/3
  DCM_w_b/1 -> DCM*I_w*Ωdot/1, DCM*I_w*Ω/1
  DCM_w_b1/1 -> DCM*I_w*Ωdot/2, DCM*I_w*Ω/2
  inv(I_b)/1 -> ω_dot = inv(I_b)*[-cross(ω,DCM*I_w*Ω)-DCM*I_w*Ωdot-cross(ω,I_b*ω)]/1
  Add/1 -> ω_dot = inv(I_b)*[-cross(ω,DCM*I_w*Ω)-DCM*I_w*Ωdot-cross(ω,I_b*ω)]/2
  DCM*I_w*Ω/1 -> cross(ω,DCM*I_w*Ω)/2
  DCM*I_w*Ωdot/1 -> Add/2
  cross(ω,DCM*I_w*Ω)/1 -> Add/1
  I_b*ω/1 -> cross(ω,I_b*ω)/2
  ω_dot = inv(I_b)*[-cross(ω,DCM*I_w*Ω)-DCM*I_w*Ωdot-cross(ω,I_b*ω)]/1 -> ω_dot/1
  ω_b/1 -> cross(ω,DCM*I_w*Ω)/1, cross(ω,I_b*ω)/1, I_b*ω/2
  cross(ω,I_b*ω)/1 -> Add/3
  DCM_w_b2/1 -> I_b*ω/1, inv(I_b)/1

== system satellite_attitude_kalman_model/air bearing/ω to DCM ==
  ω : Inport
  Constant : Constant  Value=dt_w
  Gain : Gain  Gain=-1
  Interpreted MATLAB Function : MATLABFcn  MATLABFcn=Smtrx  OutputDimensions=[3,3]  Output1D=off
  Interpreted MATLAB Function1 : MATLABFcn  MATLABFcn=expm  OutputDimensions=[3,3]  Output1D=off
  Matrix Multiply : Product  Multiplication=Matrix(*)
  Product : Product
  Unit Delay : UnitDelay  InitialCondition=DCM_b_i_0  SampleTime=-1
  Zero-Order Hold : ZeroOrderHold  SampleTime=dt_w
  DCM_b_i : Outport
  wires:
  ω/1 -> Zero-Order Hold/1
  Zero-Order Hold/1 -> Product/2
  Constant/1 -> Product/1
  Product/1 -> Interpreted MATLAB Function/1
  Interpreted MATLAB Function/1 -> Gain/1
  Gain/1 -> Interpreted MATLAB Function1/1
  Matrix Multiply/1 -> Unit Delay/1, DCM_b_i/1
  Interpreted MATLAB Function1/1 -> Matrix Multiply/1
  Unit Delay/1 -> Matrix Multiply/2

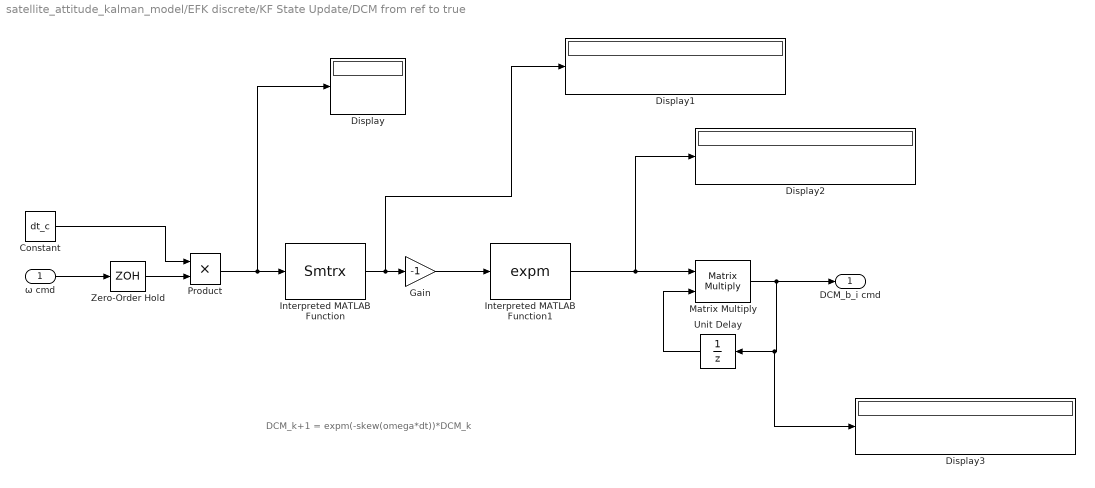
== system satellite_attitude_kalman_model/EFK discrete/KF State Update/DCM from ref to true ==
  note: DCM_k+1 = expm(-skew(omega*dt))*DCM_k
  ω cmd : Inport
  Constant : Constant  Value=dt_c
  Display{,1..3} (4 alike) : Display
  Gain : Gain  Gain=-1
  Interpreted MATLAB Function : MATLABFcn  MATLABFcn=Smtrx  OutputDimensions=[3,3]  Output1D=off
  Interpreted MATLAB Function1 : MATLABFcn  MATLABFcn=expm  OutputDimensions=[3,3]  Output1D=off
  Matrix Multiply : Product  Multiplication=Matrix(*)
  Product : Product
  Unit Delay : UnitDelay  InitialCondition=DCM_b_i_0  SampleTime=dt_c
  Zero-Order Hold : ZeroOrderHold  SampleTime=dt_c
  DCM_b_i cmd : Outport
  wires:
  ω cmd/1 -> Zero-Order Hold/1
  Zero-Order Hold/1 -> Product/2
  Constant/1 -> Product/1
  Product/1 -> Display/1, Interpreted MATLAB Function/1
  Interpreted MATLAB Function/1 -> Display1/1, Gain/1
  Gain/1 -> Interpreted MATLAB Function1/1
  Matrix Multiply/1 -> Display3/1, Unit Delay/1, DCM_b_i cmd/1
  Interpreted MATLAB Function1/1 -> Display2/1, Matrix Multiply/1
  Unit Delay/1 -> Matrix Multiply/2

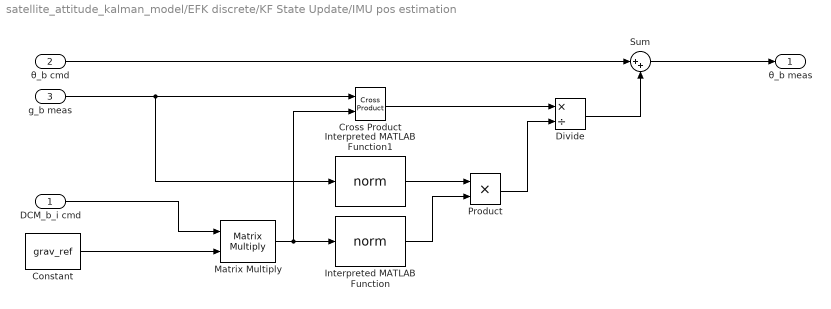
== system satellite_attitude_kalman_model/EFK discrete/KF State Update/IMU pos estimation ==
  DCM_b_i cmd : Inport
  θ_b cmd : Inport  Port=2
  g_b meas : Inport  Port=3
  Constant : Constant  Value=grav_ref  VectorParams1D=off  SampleTime=dt_c
  Cross Product : vrlib/Utilities/Cross Product
      settings: SourceProductBaseCode=VR
  Divide : Product  Inputs=*/
  Interpreted MATLAB Function : MATLABFcn  MATLABFcn=norm
  Interpreted MATLAB Function1 : MATLABFcn  MATLABFcn=norm
  Matrix Multiply : Product  Multiplication=Matrix(*)
  Product : Product
  Sum : Sum  Inputs=|++
  θ_b meas : Outport
  wires:
  Interpreted MATLAB Function/1 -> Product/2
  Divide/1 -> Sum/2
  Cross Product/1 -> Divide/1
  Product/1 -> Divide/2
  Constant/1 -> Matrix Multiply/2
  Matrix Multiply/1 -> Interpreted MATLAB Function/1, Cross Product/2
  θ_b cmd/1 -> Sum/1
  g_b meas/1 -> Interpreted MATLAB Function1/1, Cross Product/1
  DCM_b_i cmd/1 -> Matrix Multiply/1
  Sum/1 -> θ_b meas/1
  Interpreted MATLAB Function1/1 -> Product/1

== system satellite_attitude_kalman_model/EFK discrete/KF State Update/MAG pos estimation ==
  DCM cmd : Inport
  θ cmd : Inport  Port=2
  m meas : Inport  Port=3
  Constant : Constant  Value=mag_ref  VectorParams1D=off  SampleTime=dt_c
  Cross Product : vrlib/Utilities/Cross Product
      settings: SourceProductBaseCode=VR
  Divide : Product  Inputs=*/
  Interpreted MATLAB Function : MATLABFcn  MATLABFcn=norm  Output1D=off
  Interpreted MATLAB Function1 : MATLABFcn  MATLABFcn=norm  Output1D=off
  Matrix Multiply : Product  Multiplication=Matrix(*)
  Product : Product
  Sum : Sum  Inputs=|++
  θ_b meas : Outport
  wires:
  Interpreted MATLAB Function/1 -> Product/2
  Divide/1 -> Sum/2
  Cross Product/1 -> Divide/1
  Product/1 -> Divide/2
  Constant/1 -> Matrix Multiply/2
  Matrix Multiply/1 -> Interpreted MATLAB Function/1, Cross Product/2
  θ cmd/1 -> Sum/1
  m meas/1 -> Interpreted MATLAB Function1/1, Cross Product/1
  DCM cmd/1 -> Matrix Multiply/1
  Sum/1 -> θ_b meas/1
  Interpreted MATLAB Function1/1 -> Product/1
